simulink model "STOICAL_example_2_Step01_ModelExtension"  (R2014b)
settings: Solver=ode4  StartTime=0.0  StopTime=1  FixedStep=50E-6  RelTol=1e-3
model workspace (MAT data in the model file):
  STOVICAL.SignalSaveOptions.ReturnWorkspaceOutputs = 'on'
  STOVICAL.SignalSaveOptions.ReturnWorkspaceOutputsName = 'simout_obj'
  STOVICAL.SignalSaveOptions.SignalLogging = 'on'
  STOVICAL.SignalSaveOptions.SignalLoggingSaveFormat = 'Dataset'
  STOVICAL.SignalSaveOptions.SignalLoggingName = 'STOVICAL_LoggedSignals'
  STOVICAL.ParameterDefinition.BlkNameFull{1} = 'Step amplitude
    | #PARAM#Amplitude'
  STOVICAL.ParameterDefinition.BlkNameFull{2} = 'Static System
    | modelled
    | by gain block
    | #PARAM#SystemGain'
  STOVICAL.ParameterDefinition.BlkNameShort{1} = 'Step amplitude
    | '
  STOVICAL.ParameterDefinition.BlkNameShort{2} = 'Static System
    | modelled
    | by gain block
    | '
  STOVICAL.ParameterDefinition.BlkHandle = [1972.00012207; 1979.00012207]
  STOVICAL.ParameterDefinition.ParamName = {'Amplitude'; 'SystemGain'}
  STOVICAL.ParameterDefinition.BlkPath{1} = 'STOICAL_example_1_Step02b_ActivateParameters/#UNIT#Stimulus/Step amplitude
    | #PARAM#Amplitude'
  STOVICAL.ParameterDefinition.BlkPath{2} = 'STOICAL_example_1_Step02b_ActivateParameters/#UNIT#System/Static System
    | modelled
    | by gain block
    | #PARAM#SystemGain'
  STOVICAL.ParameterDefinition.BlkType = {'Constant'; 'Gain'}
  STOVICAL.ParameterDefinition.BlkMaskType = {''; ''}
  STOVICAL.ParameterDefinition.ParentalBlockPath = {'STOICAL_example_1_Step02b_ActivateParameters/#UNIT#Stimulus'; 'STOICAL_example_1_Step02b_ActivateParameters/#UNIT#System'}
  STOVICAL.ParameterDefinition.ParentalBlockHandle = [1969.00012207; 1977.00036621]
  STOVICAL.ParameterDefinition.Belongs2SubsystemHdl = [1969.00012207; 1977.00036621]
  STOVICAL.ParameterDefinition.NrParams = 2
  STOVICAL.ParameterDefinition.BlkField2Set = {'Value'; 'Gain'}
  STOVICAL.ParameterDefinition.BlkFieldSyntax = {'#'; '#'}
  STOVICAL.ParameterDefinition.ParamVariable = {'param_ec6e274da2c23e664dfdc874ac252818'; 'param_afc1e04cc1c158b687408e5b6ea19d06'}
  STOVICAL.ParameterDefinition.LabelPath = {'#Stimulus#Amplitude'; '#System#SystemGain'}
  STOVICAL.ParameterDefinition.ParamDefaultValue = {'2'; '5'}
  STOVICAL.SignalDefinition.ParentalBlockPath = {'STOICAL_example_1_Step02c_ActivateSignals'; 'STOICAL_example_1_Step02c_ActivateSignals'}
  STOVICAL.SignalDefinition.ParentalBlockHandle = [1967.00048828; 1967.00048828]
  STOVICAL.SignalDefinition.NameInDiagram = {'#SIG#stimulus'; '#SIG#response'}
  STOVICAL.SignalDefinition.SourceBlockPath = {'STOICAL_example_1_Step02c_ActivateSignals/#UNIT#Stimulus'; 'STOICAL_example_1_Step02c_ActivateSignals/#UNIT#System'}
  STOVICAL.SignalDefinition.SourceBlockPort = [1; 1]
  STOVICAL.SignalDefinition.SourceBlockHandle = [1969.00195312; 1977.00073242]
  STOVICAL.SignalDefinition.Handle = [1988.00097656; 1989.00073242]
  STOVICAL.SignalDefinition.NrSig = 2
  STOVICAL.SignalDefinition.NameOfLogVar = {'logsig_47c2411a71c8218b6c2a20514199b03d'; 'logsig_5069e1d9063564028bd2189e4cf0bc84'}
  STOVICAL.SignalDefinition.NameOfLogVarMode = {'SignalName'; 'SignalName'}
  STOVICAL.SignalDefinition.DoLog = [0; 0]
  STOVICAL.SignalDefinition.LabelPath = {'#stimulus'; '#response'}
  STOVICAL.VariantDefinition.NodeHandle = [1967.00073242; 1969.00561523; 1977.00146484]
  STOVICAL.VariantDefinition.NodeName = {'STOICAL_example_1_Step02d_ActivateVariants'; '#UNIT#Stimulus'; '#UNIT#System'}
  STOVICAL.VariantDefinition.IsVariantSubsystem = [0; 0; 0]
  STOVICAL.VariantDefinition.NodeLevel = [1; 2; 2]
  STOVICAL.VariantDefinition.NodePath = {'STOICAL_example_1_Step02d_ActivateVariants'; 'STOICAL_example_1_Step02d_ActivateVariants/#UNIT#Stimulus'; 'STOICAL_example_1_Step02d_ActivateVariants/#UNIT#System'}
  STOVICAL.VariantDefinition.IsVariant = [0; 0; 0]
  STOVICAL.VariantDefinition.VSNodeIdxofVariant = [0; 0; 0]
  STOVICAL.VariantDefinition.VSVariantsCount = [0; 0; 0]
  STOVICAL.VariantDefinition.VSVariantsBlkHdls = {[]; []; []}
  STOVICAL.VariantDefinition.VSVariantsNodeIdx = {[]; []; []}
  STOVICAL.VariantDefinition.VSControlVariable = {[]; []; []}
  STOVICAL.VariantDefinition.VSVariantHasNr = [0; 0; 0]
  STOVICAL.VariantDefinition.LabelPath = {[]; []; []}
  param_ec6e274da2c23e664dfdc874ac252818 = '2'
  param_afc1e04cc1c158b687408e5b6ea19d06 = '5'
settings Model: Creator=Wippenbeck  LastModifiedBy=Wippenbeck
settings DataIOCC: ReturnWorkspaceOutputs=on  SignalLoggingName=STOVICAL_LoggedSignals  ReturnWorkspaceOutputsName=simout_obj

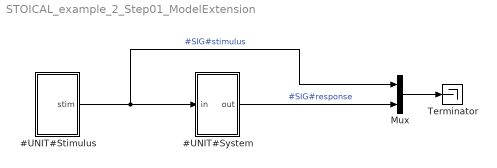
== system STOICAL_example_2_Step01_ModelExtension ==
  #UNIT#Stimulus : Subsystem
  #UNIT#System : Subsystem
  Mux : Mux  Inputs=2
  Terminator : Terminator
  wires:
  Mux/1 -> Terminator/1
  #UNIT#Stimulus/1(stim) -> #UNIT#System/1(in), Mux/1  "#SIG#stimulus"
  #UNIT#System/1(out) -> Mux/2  "#SIG#response"

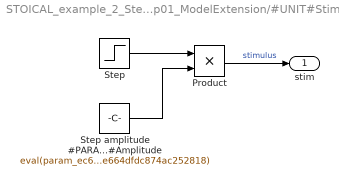
== system STOICAL_example_2_Step01_ModelExtension/#UNIT#Stimulus ==
  Product : Product
  Step : Step  Time=0.1  SampleTime=0
  Step amplitude #PARAM#Amplitude : Constant  Value=eval(param_ec6e274da2c23e664dfdc874ac252818)
  stim : Outport
  wires:
  Step amplitude #PARAM#Amplitude/1 -> Product/2
  Product/1 -> stim/1  "stimulus"
  Step/1 -> Product/1

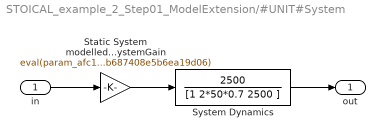
== system STOICAL_example_2_Step01_ModelExtension/#UNIT#System ==
  in : Inport
  Static System modelled by gain block #PARAM#SystemGain : Gain  Gain=eval(param_afc1e04cc1c158b687408e5b6ea19d06)
  System Dynamics : TransferFcn  Numerator=[2500]  Denominator=[1 2*50*0.7 2500 ]
  out : Outport
  wires:
  Static System modelled by gain block #PARAM#SystemGain/1 -> System Dynamics/1
  in/1 -> Static System modelled by gain block #PARAM#SystemGain/1
  System Dynamics/1 -> out/1
